simulink model "demo_duffing"  (Simulink 2.20)
settings: Solver=ode45  StartTime=0.0  StopTime=5.0  RelTol=1e-3  AbsTol=1e-6
libraries: NelinSys x2
settings Model: ConsistencyChecking=off  RTWPlaceOutputsASAP=off

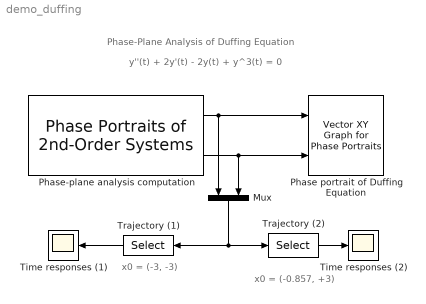
== system demo_duffing ==
  note: Phase-Plane Analysis of Duffing Equation
  note: y''(t) + 2y'(t) - 2y(t) + y^3(t) = 0
  note: x0 = (-3, -3)
  note: x0 = (-0.857, +3)
  Mux : Mux  Orientation=down  Inputs=2
  Phase portrait of Duffing Equation : NelinSys/Nonlinear Systems Analysis/Vector XY Graph for Phase Portraits  xmin=-4  xmax=4  ymin=-4  ymax=4  st=-1  use_grid=on
  Phase-plane analysis computation : NelinSys/Nonlinear Systems Analysis/Phase Portraits of 2nd-Order Systems  vRovnica=D2y+2*Dy-2*y+y^3=0  x1min=-3  x1max=3  x1num=15  x2min=-3  x2max=3  x2num=3
  Time responses (1) : Scope
      settings: TickLabels=on  TimeRange=auto  YMin=-4  YMax=4  SaveToWorkspace=off  SaveName=ScopeData
  Time responses (2) : Scope
      settings: TickLabels=on  TimeRange=auto  YMin=-1  YMax=3  SaveToWorkspace=off  SaveName=ScopeData
  Trajectory (1) : Selector  Orientation=left  Elements=[1 46]  InputPortWidth=90
  Trajectory (2) : Selector  Elements=[18 63]  InputPortWidth=90
  wires:
  Trajectory (2)/1 -> Time responses (2)/1
  Trajectory (1)/1 -> Time responses (1)/1
  Mux/1 -> Trajectory (2)/1, Trajectory (1)/1
  Phase-plane analysis computation/1 -> Phase portrait of Duffing Equation/1, Mux/1
  Phase-plane analysis computation/2 -> Phase portrait of Duffing Equation/2, Mux/2
